simulink model "gm_Model"  (R2025a)
settings: Solver=FixedStepDiscrete  StartTime=0.0  StopTime=80000/fs_in  RelTol=1e-3
undefined symbols (not defined in the file or in its folder): a, b, b_fixp, beta_retanh, c, cos_omega, cos_omega_fixp, diag_count, exp_omega, exp_omega_fixp, fixp_chebacc_frac, fixp_chebacc_ws, fixp_dsp_ws, fixp_eig_frac, fixp_eig_ws, fs_in, group_size, hann_table_fixp, image_seed, image_seed_fixp, J_ROM, k, K_ROM, lap_diags, lap_main, lap_main_fi, lap_offsets, lap_offsets_fi, lap_rest, lap_rest_fi, laplacian_diags_main, laplacian_diags_offsets, laplacian_diags_rest, lut_norm_x, lut_norm_y, magnitude, n_ch, n_layer, n_px, n_px_fi, nf, norm_gain_floor, power_iters, power_norm_scaling_factor_fixp, tau, tau_fixp, theta, theta_fixp
libraries: simulink x59, hdlsllib x36, hdlstreaminglib x4, hdlmdlgenlib x1, matrix_library x1, dspvision x1
(part 6 of 8)

== system gm_Model/DUT_Test/Goertzel/EnabledGoertzel/streaming_partition_streamed1 ==
  in0 : Inport  OutDataTypeStr=fixdt(1, 18, 13)  PortDimensions=[1 48]  SampleTime=3.125e-07
      settings: SignalType=complex
  in1 : Inport  Port=2  OutDataTypeStr=boolean  SampleTime=3.125e-07
  in2 : Inport  Port=3  OutDataTypeStr=fixdt(1, 18, 13)  PortDimensions=[1 48]  SampleTime=3.125e-07
      settings: SignalType=complex
  enb_counter : Inport  Port=4  OutDataTypeStr=uint8  SampleTime=3.125e-07
  Delay3_enbsw : Switch  Criteria=u2 ~= 0  Threshold=double(0)  OutDataTypeStr=fixdt(1, 18, 13)  SampleTime=3.125e-07  SaturateOnIntegerOverflow=off  InputSameDT=off
  Serializer_Subnetwork : Subsystem
  Serializer_Subnetwork1 : Subsystem
  Sum of Elements_out1_bypass : Subsystem
  counter : Subsystem
  enb_counter_eq_97 : simulink/Logic and Bit Operations/Compare To Constant  relop===  const=double(97)  OutDataTypeStr=boolean
  enb_counter_ge_50 : simulink/Logic and Bit Operations/Compare To Constant  relop=>=  const=double(50)  OutDataTypeStr=boolean
  enb_counter_ge_50_and_enb_counter_le_96 : Logic  AllPortsSameDT=off  OutDataTypeStr=boolean  SampleTime=3.125e-07
  enb_counter_le_47 : simulink/Logic and Bit Operations/Compare To Constant  relop=<=  const=double(47)  OutDataTypeStr=boolean
  enb_counter_le_96 : simulink/Logic and Bit Operations/Compare To Constant  relop=<=  const=double(96)  OutDataTypeStr=boolean
  rd_{0..1,3..4,7..8,10..11} (8 alike) : Delay  DelayLength=double(1)  InitialCondition=0  SampleTime=3.125e-07
  rd_12 : Delay  DelayLength=double(6)  InitialCondition=0  SampleTime=3.125e-07
  rd_2 : Delay  DelayLength=double(53)  InitialCondition=0  SampleTime=3.125e-07
  rd_5 : Delay  DelayLength=double(55)  InitialCondition=0  SampleTime=3.125e-07
  rd_6 : Delay  DelayLength=double(54)  InitialCondition=0  SampleTime=3.125e-07
  rd_9 : Delay  DelayLength=double(4)  InitialCondition=0  SampleTime=3.125e-07
  t : Mux  Inputs=2
  tappedDelay : Subsystem
  out0 : Outport  OutDataTypeStr=fixdt(1, 18, 13)  PortDimensions=[1 48]  SampleTime=3.125e-07
      settings: SignalType=complex
  wires:
  rd_3/1 -> Delay3_enbsw/1
  enb_counter/1 -> enb_counter_eq_97/1, enb_counter_le_96/1, enb_counter_ge_50/1, enb_counter_le_47/1
  rd_8/1 -> enb_counter_ge_50_and_enb_counter_le_96/2
  enb_counter_ge_50/1 -> rd_7/1
  enb_counter_le_96/1 -> rd_8/1
  enb_counter_le_47/1 -> rd_1/1
  in0/1 -> rd_0/1
  rd_7/1 -> enb_counter_ge_50_and_enb_counter_le_96/1
  in2/1 -> rd_4/1
  tappedDelay/1(out0) -> rd_10/1
  rd_1/1 -> counter/Enable
  t/1 -> out0/1
  enb_counter_ge_50_and_enb_counter_le_96/1 -> rd_9/1
  rd_5/1 -> Delay3_enbsw/2
  rd_4/1 -> Serializer_Subnetwork1/1(in0)
  counter/1(out0) -> rd_2/1, Serializer_Subnetwork1/2(in1)
  rd_0/1 -> Serializer_Subnetwork/1(in0)
  rd_6/1 -> Delay3_enbsw/3
  rd_2/1 -> Serializer_Subnetwork/2(in1)
  Serializer_Subnetwork/1(out0) -> rd_3/1
  Serializer_Subnetwork1/1(out0) -> rd_6/1
  Delay3_enbsw/1 -> rd_11/1, tappedDelay/1(in0)
  enb_counter_eq_97/1 -> rd_12/1
  rd_12/1 -> Sum of Elements_out1_bypass/2(in1)
  in1/1 -> rd_5/1
  rd_9/1 -> tappedDelay/Enable
  rd_11/1 -> Sum of Elements_out1_bypass/1(in0)
  rd_10/1 -> t/1
  Sum of Elements_out1_bypass/1(out0) -> t/2

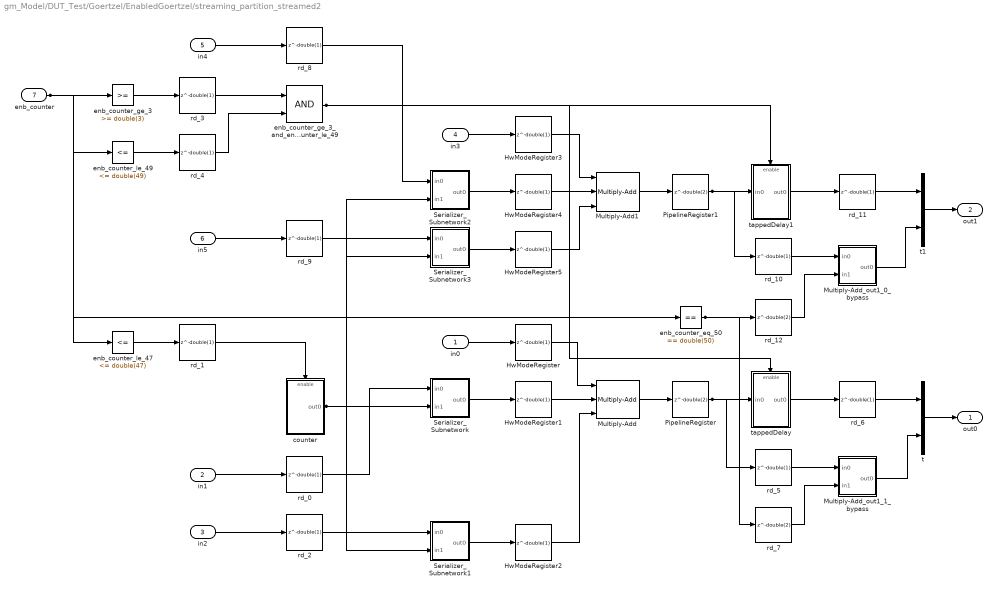
== system gm_Model/DUT_Test/Goertzel/EnabledGoertzel/streaming_partition_streamed2 ==
  in0 : Inport  OutDataTypeStr=fixdt(1, 18, 13)  SampleTime=3.125e-07
      settings: SignalType=complex
  in1 : Inport  Port=2  OutDataTypeStr=fixdt(1, 18, 13)  PortDimensions=[1 48]  SampleTime=3.125e-07
  in2 : Inport  Port=3  OutDataTypeStr=fixdt(1, 18, 13)  PortDimensions=[1 48]  SampleTime=3.125e-07
  in3 : Inport  Port=4  OutDataTypeStr=fixdt(1, 18, 13)  SampleTime=3.125e-07
      settings: SignalType=complex
  in4 : Inport  Port=5  OutDataTypeStr=fixdt(1, 18, 13)  PortDimensions=[1 48]  SampleTime=3.125e-07
  in5 : Inport  Port=6  OutDataTypeStr=fixdt(1, 18, 13)  PortDimensions=[1 48]  SampleTime=3.125e-07
  enb_counter : Inport  Port=7  OutDataTypeStr=uint8  SampleTime=3.125e-07
  HwModeRegister{,1..5} (6 alike) : Delay  DelayLength=double(1)  InitialCondition=0  SampleTime=3.125e-07
  Multiply-Add : hdlsllib/HDL Operations/Multiply-Add  Function=c-(a.*b)  datatype=fixdt(1, 18, 13)  DoSatur=off  FMA=off
  Multiply-Add1 : hdlsllib/HDL Operations/Multiply-Add  Function=c-(a.*b)  datatype=fixdt(1, 18, 13)  DoSatur=off  FMA=off
  Multiply-Add_out1_0_bypass : Subsystem
  Multiply-Add_out1_1_bypass : Subsystem
  PipelineRegister : Delay  DelayLength=double(2)  InitialCondition=0  SampleTime=3.125e-07
  PipelineRegister1 : Delay  DelayLength=double(2)  InitialCondition=0  SampleTime=3.125e-07
  Serializer_Subnetwork : Subsystem
  Serializer_Subnetwork1 : Subsystem
  Serializer_Subnetwork2 : Subsystem
  Serializer_Subnetwork3 : Subsystem
  counter : Subsystem
  enb_counter_eq_50 : simulink/Logic and Bit Operations/Compare To Constant  relop===  const=double(50)  OutDataTypeStr=boolean
  enb_counter_ge_3 : simulink/Logic and Bit Operations/Compare To Constant  relop=>=  const=double(3)  OutDataTypeStr=boolean
  enb_counter_ge_3_and_enb_counter_le_49 : Logic  AllPortsSameDT=off  OutDataTypeStr=boolean  SampleTime=3.125e-07
  enb_counter_le_47 : simulink/Logic and Bit Operations/Compare To Constant  relop=<=  const=double(47)  OutDataTypeStr=boolean
  enb_counter_le_49 : simulink/Logic and Bit Operations/Compare To Constant  relop=<=  const=double(49)  OutDataTypeStr=boolean
  rd_{0..6,8..11} (11 alike) : Delay  DelayLength=double(1)  InitialCondition=0  SampleTime=3.125e-07
  rd_12 : Delay  DelayLength=double(2)  InitialCondition=0  SampleTime=3.125e-07
  rd_7 : Delay  DelayLength=double(2)  InitialCondition=0  SampleTime=3.125e-07
  t : Mux  Inputs=2
  t1 : Mux  Inputs=2
  tappedDelay : Subsystem
  tappedDelay1 : Subsystem
  out0 : Outport  OutDataTypeStr=fixdt(1, 18, 13)  PortDimensions=[1 48]  SampleTime=3.125e-07
      settings: SignalType=complex
  out1 : Outport  Port=2  OutDataTypeStr=fixdt(1, 18, 13)  PortDimensions=[1 48]  SampleTime=3.125e-07
      settings: SignalType=complex
  wires:
  tappedDelay/1(out0) -> rd_6/1
  enb_counter_le_49/1 -> rd_4/1
  HwModeRegister/1 -> Multiply-Add/1
  enb_counter/1 -> enb_counter_le_49/1, enb_counter_ge_3/1, enb_counter_le_47/1, enb_counter_eq_50/1
  rd_4/1 -> enb_counter_ge_3_and_enb_counter_le_49/2
  rd_5/1 -> Multiply-Add_out1_1_bypass/1(in0)
  Serializer_Subnetwork3/1(out0) -> HwModeRegister5/1
  in1/1 -> rd_0/1
  rd_3/1 -> enb_counter_ge_3_and_enb_counter_le_49/1
  enb_counter_ge_3/1 -> rd_3/1
  enb_counter_le_47/1 -> rd_1/1
  rd_12/1 -> Multiply-Add_out1_0_bypass/2(in1)
  in5/1 -> rd_9/1
  in4/1 -> rd_8/1
  rd_1/1 -> counter/Enable
  in2/1 -> rd_2/1
  rd_8/1 -> Serializer_Subnetwork2/1(in0)
  enb_counter_ge_3_and_enb_counter_le_49/1 -> tappedDelay1/Enable, tappedDelay/Enable
  rd_2/1 -> Serializer_Subnetwork1/1(in0)
  rd_9/1 -> Serializer_Subnetwork3/1(in0)
  counter/1(out0) -> Serializer_Subnetwork3/2(in1), Serializer_Subnetwork2/2(in1), Serializer_Subnetwork1/2(in1), Serializer_Subnetwork/2(in1)
  in0/1 -> HwModeRegister/1
  rd_0/1 -> Serializer_Subnetwork/1(in0)
  in3/1 -> HwModeRegister3/1
  Serializer_Subnetwork2/1(out0) -> HwModeRegister4/1
  Serializer_Subnetwork/1(out0) -> HwModeRegister1/1
  HwModeRegister5/1 -> Multiply-Add1/3
  HwModeRegister3/1 -> Multiply-Add1/1
  Serializer_Subnetwork1/1(out0) -> HwModeRegister2/1
  HwModeRegister4/1 -> Multiply-Add1/2
  PipelineRegister1/1 -> rd_10/1, tappedDelay1/1(in0)
  Multiply-Add/1 -> PipelineRegister/1
  HwModeRegister1/1 -> Multiply-Add/2
  HwModeRegister2/1 -> Multiply-Add/3
  Multiply-Add1/1 -> PipelineRegister1/1
  Multiply-Add_out1_1_bypass/1(out0) -> t/2
  enb_counter_eq_50/1 -> rd_7/1, rd_12/1
  PipelineRegister/1 -> rd_5/1, tappedDelay/1(in0)
  tappedDelay1/1(out0) -> rd_11/1
  rd_10/1 -> Multiply-Add_out1_0_bypass/1(in0)
  rd_7/1 -> Multiply-Add_out1_1_bypass/2(in1)
  rd_6/1 -> t/1
  rd_11/1 -> t1/1
  Multiply-Add_out1_0_bypass/1(out0) -> t1/2
  t1/1 -> out1/1
  t/1 -> out0/1

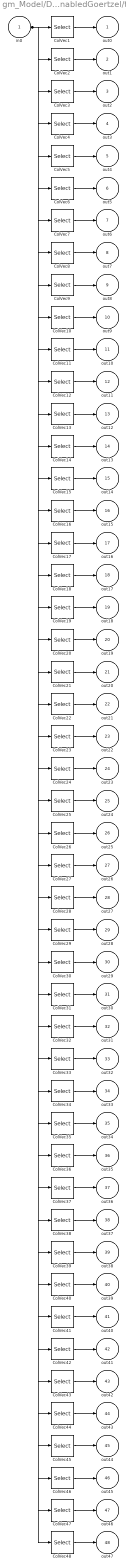
== system gm_Model/DUT_Test/Goertzel/EnabledGoertzel/t2 ==
  in0 : Inport
  ColVec1 : Selector  NumberOfDimensions=2  IndexOptions=Select all,Index vector (dialog)  Indices=1,1  OutputSizes=1,1
  ColVec10 : Selector  NumberOfDimensions=2  IndexOptions=Select all,Index vector (dialog)  Indices=1,10  OutputSizes=1,1
  ColVec11 : Selector  NumberOfDimensions=2  IndexOptions=Select all,Index vector (dialog)  Indices=1,11  OutputSizes=1,1
  ColVec12 : Selector  NumberOfDimensions=2  IndexOptions=Select all,Index vector (dialog)  Indices=1,12  OutputSizes=1,1
  ColVec13 : Selector  NumberOfDimensions=2  IndexOptions=Select all,Index vector (dialog)  Indices=1,13  OutputSizes=1,1
  ColVec14 : Selector  NumberOfDimensions=2  IndexOptions=Select all,Index vector (dialog)  Indices=1,14  OutputSizes=1,1
  ColVec15 : Selector  NumberOfDimensions=2  IndexOptions=Select all,Index vector (dialog)  Indices=1,15  OutputSizes=1,1
  ColVec16 : Selector  NumberOfDimensions=2  IndexOptions=Select all,Index vector (dialog)  Indices=1,16  OutputSizes=1,1
  ColVec17 : Selector  NumberOfDimensions=2  IndexOptions=Select all,Index vector (dialog)  Indices=1,17  OutputSizes=1,1
  ColVec18 : Selector  NumberOfDimensions=2  IndexOptions=Select all,Index vector (dialog)  Indices=1,18  OutputSizes=1,1
  ColVec19 : Selector  NumberOfDimensions=2  IndexOptions=Select all,Index vector (dialog)  Indices=1,19  OutputSizes=1,1
  ColVec2 : Selector  NumberOfDimensions=2  IndexOptions=Select all,Index vector (dialog)  Indices=1,2  OutputSizes=1,1
  ColVec20 : Selector  NumberOfDimensions=2  IndexOptions=Select all,Index vector (dialog)  Indices=1,20  OutputSizes=1,1
  ColVec21 : Selector  NumberOfDimensions=2  IndexOptions=Select all,Index vector (dialog)  Indices=1,21  OutputSizes=1,1
  ColVec22 : Selector  NumberOfDimensions=2  IndexOptions=Select all,Index vector (dialog)  Indices=1,22  OutputSizes=1,1
  ColVec23 : Selector  NumberOfDimensions=2  IndexOptions=Select all,Index vector (dialog)  Indices=1,23  OutputSizes=1,1
  ColVec24 : Selector  NumberOfDimensions=2  IndexOptions=Select all,Index vector (dialog)  Indices=1,24  OutputSizes=1,1
  ColVec25 : Selector  NumberOfDimensions=2  IndexOptions=Select all,Index vector (dialog)  Indices=1,25  OutputSizes=1,1
  ColVec26 : Selector  NumberOfDimensions=2  IndexOptions=Select all,Index vector (dialog)  Indices=1,26  OutputSizes=1,1
  ColVec27 : Selector  NumberOfDimensions=2  IndexOptions=Select all,Index vector (dialog)  Indices=1,27  OutputSizes=1,1
  ColVec28 : Selector  NumberOfDimensions=2  IndexOptions=Select all,Index vector (dialog)  Indices=1,28  OutputSizes=1,1
  ColVec29 : Selector  NumberOfDimensions=2  IndexOptions=Select all,Index vector (dialog)  Indices=1,29  OutputSizes=1,1
  ColVec3 : Selector  NumberOfDimensions=2  IndexOptions=Select all,Index vector (dialog)  Indices=1,3  OutputSizes=1,1
  ColVec30 : Selector  NumberOfDimensions=2  IndexOptions=Select all,Index vector (dialog)  Indices=1,30  OutputSizes=1,1
  ColVec31 : Selector  NumberOfDimensions=2  IndexOptions=Select all,Index vector (dialog)  Indices=1,31  OutputSizes=1,1
  ColVec32 : Selector  NumberOfDimensions=2  IndexOptions=Select all,Index vector (dialog)  Indices=1,32  OutputSizes=1,1
  ColVec33 : Selector  NumberOfDimensions=2  IndexOptions=Select all,Index vector (dialog)  Indices=1,33  OutputSizes=1,1
  ColVec34 : Selector  NumberOfDimensions=2  IndexOptions=Select all,Index vector (dialog)  Indices=1,34  OutputSizes=1,1
  ColVec35 : Selector  NumberOfDimensions=2  IndexOptions=Select all,Index vector (dialog)  Indices=1,35  OutputSizes=1,1
  ColVec36 : Selector  NumberOfDimensions=2  IndexOptions=Select all,Index vector (dialog)  Indices=1,36  OutputSizes=1,1
  ColVec37 : Selector  NumberOfDimensions=2  IndexOptions=Select all,Index vector (dialog)  Indices=1,37  OutputSizes=1,1
  ColVec38 : Selector  NumberOfDimensions=2  IndexOptions=Select all,Index vector (dialog)  Indices=1,38  OutputSizes=1,1
  ColVec39 : Selector  NumberOfDimensions=2  IndexOptions=Select all,Index vector (dialog)  Indices=1,39  OutputSizes=1,1
  ColVec4 : Selector  NumberOfDimensions=2  IndexOptions=Select all,Index vector (dialog)  Indices=1,4  OutputSizes=1,1
  ColVec40 : Selector  NumberOfDimensions=2  IndexOptions=Select all,Index vector (dialog)  Indices=1,40  OutputSizes=1,1
  ColVec41 : Selector  NumberOfDimensions=2  IndexOptions=Select all,Index vector (dialog)  Indices=1,41  OutputSizes=1,1
  ColVec42 : Selector  NumberOfDimensions=2  IndexOptions=Select all,Index vector (dialog)  Indices=1,42  OutputSizes=1,1
  ColVec43 : Selector  NumberOfDimensions=2  IndexOptions=Select all,Index vector (dialog)  Indices=1,43  OutputSizes=1,1
  ColVec44 : Selector  NumberOfDimensions=2  IndexOptions=Select all,Index vector (dialog)  Indices=1,44  OutputSizes=1,1
  ColVec45 : Selector  NumberOfDimensions=2  IndexOptions=Select all,Index vector (dialog)  Indices=1,45  OutputSizes=1,1
  ColVec46 : Selector  NumberOfDimensions=2  IndexOptions=Select all,Index vector (dialog)  Indices=1,46  OutputSizes=1,1
  ColVec47 : Selector  NumberOfDimensions=2  IndexOptions=Select all,Index vector (dialog)  Indices=1,47  OutputSizes=1,1
  ColVec48 : Selector  NumberOfDimensions=2  IndexOptions=Select all,Index vector (dialog)  Indices=1,48  OutputSizes=1,1
  ColVec5 : Selector  NumberOfDimensions=2  IndexOptions=Select all,Index vector (dialog)  Indices=1,5  OutputSizes=1,1
  ColVec6 : Selector  NumberOfDimensions=2  IndexOptions=Select all,Index vector (dialog)  Indices=1,6  OutputSizes=1,1
  ColVec7 : Selector  NumberOfDimensions=2  IndexOptions=Select all,Index vector (dialog)  Indices=1,7  OutputSizes=1,1
  ColVec8 : Selector  NumberOfDimensions=2  IndexOptions=Select all,Index vector (dialog)  Indices=1,8  OutputSizes=1,1
  ColVec9 : Selector  NumberOfDimensions=2  IndexOptions=Select all,Index vector (dialog)  Indices=1,9  OutputSizes=1,1
  out0 : Outport
  out1 : Outport  Port=2
  out2 : Outport  Port=3
  out3 : Outport  Port=4
  out4 : Outport  Port=5
  out5 : Outport  Port=6
  out6 : Outport  Port=7
  out7 : Outport  Port=8
  out8 : Outport  Port=9
  out9 : Outport  Port=10
  out10 : Outport  Port=11
  out11 : Outport  Port=12
  out12 : Outport  Port=13
  out13 : Outport  Port=14
  out14 : Outport  Port=15
  out15 : Outport  Port=16
  out16 : Outport  Port=17
  out17 : Outport  Port=18
  out18 : Outport  Port=19
  out19 : Outport  Port=20
  out20 : Outport  Port=21
  out21 : Outport  Port=22
  out22 : Outport  Port=23
  out23 : Outport  Port=24
  out24 : Outport  Port=25
  out25 : Outport  Port=26
  out26 : Outport  Port=27
  out27 : Outport  Port=28
  out28 : Outport  Port=29
  out29 : Outport  Port=30
  out30 : Outport  Port=31
  out31 : Outport  Port=32
  out32 : Outport  Port=33
  out33 : Outport  Port=34
  out34 : Outport  Port=35
  out35 : Outport  Port=36
  out36 : Outport  Port=37
  out37 : Outport  Port=38
  out38 : Outport  Port=39
  out39 : Outport  Port=40
  out40 : Outport  Port=41
  out41 : Outport  Port=42
  out42 : Outport  Port=43
  out43 : Outport  Port=44
  out44 : Outport  Port=45
  out45 : Outport  Port=46
  out46 : Outport  Port=47
  out47 : Outport  Port=48
  wires:
  in0/1 -> ColVec1/1, ColVec2/1, ColVec3/1, ColVec4/1, ColVec5/1, ColVec6/1, ColVec7/1, ColVec8/1, ColVec9/1, ColVec10/1, ColVec11/1, ColVec12/1, ColVec13/1, ColVec14/1, ColVec15/1, ColVec16/1, ColVec17/1, ColVec18/1, ColVec19/1, ColVec20/1, ColVec21/1, ColVec22/1, ColVec23/1, ColVec24/1, ColVec25/1, ColVec26/1, ColVec27/1, ColVec28/1, ColVec29/1, ColVec30/1, ColVec31/1, ColVec32/1, ColVec33/1, ColVec34/1, ColVec35/1, ColVec36/1, ColVec37/1, ColVec38/1, ColVec39/1, ColVec40/1, ColVec41/1, ColVec42/1, ColVec43/1, ColVec44/1, ColVec45/1, ColVec46/1, ColVec47/1, ColVec48/1
  ColVec1/1 -> out0/1
  ColVec2/1 -> out1/1
  ColVec3/1 -> out2/1
  ColVec4/1 -> out3/1
  ColVec5/1 -> out4/1
  ColVec6/1 -> out5/1
  ColVec7/1 -> out6/1
  ColVec8/1 -> out7/1
  ColVec9/1 -> out8/1
  ColVec10/1 -> out9/1
  ColVec11/1 -> out10/1
  ColVec12/1 -> out11/1
  ColVec13/1 -> out12/1
  ColVec14/1 -> out13/1
  ColVec15/1 -> out14/1
  ColVec16/1 -> out15/1
  ColVec17/1 -> out16/1
  ColVec18/1 -> out17/1
  ColVec19/1 -> out18/1
  ColVec20/1 -> out19/1
  ColVec21/1 -> out20/1
  ColVec22/1 -> out21/1
  ColVec23/1 -> out22/1
  ColVec24/1 -> out23/1
  ColVec25/1 -> out24/1
  ColVec26/1 -> out25/1
  ColVec27/1 -> out26/1
  ColVec28/1 -> out27/1
  ColVec29/1 -> out28/1
  ColVec30/1 -> out29/1
  ColVec31/1 -> out30/1
  ColVec32/1 -> out31/1
  ColVec33/1 -> out32/1
  ColVec34/1 -> out33/1
  ColVec35/1 -> out34/1
  ColVec36/1 -> out35/1
  ColVec37/1 -> out36/1
  ColVec38/1 -> out37/1
  ColVec39/1 -> out38/1
  ColVec40/1 -> out39/1
  ColVec41/1 -> out40/1
  ColVec42/1 -> out41/1
  ColVec43/1 -> out42/1
  ColVec44/1 -> out43/1
  ColVec45/1 -> out44/1
  ColVec46/1 -> out45/1
  ColVec47/1 -> out46/1
  ColVec48/1 -> out47/1

== system gm_Model/DUT_ref/CrossCor/Grouping/DataValidDownsampler ==
  ValidFast : Inport
  DataFast : Inport  Port=2
  DataInSW : Switch  Criteria=u2 ~= 0  SaturateOnIntegerOverflow=off  InputSameDT=off
  DataMem : Delay  DelayLength=1
  DataRT : RateTransition  Deterministic=off  OutPortSampleTimeOpt=Multiple of input port sample time  OutPortSampleTimeMultiple=rate_factor
  RisingEdgeDetector : Subsystem
  Terminator : Terminator
  ValidMem : Delay  DelayLength=1  ShowEnablePort=on
      settings: InputPortMap=u0,e6
  ValidRT : RateTransition  Deterministic=off  OutPortSampleTimeOpt=Multiple of input port sample time  OutPortSampleTimeMultiple=rate_factor
  ValidResetCounter : hdlsllib/Sources/HDL Counter  CountType=Count limited  CountInit=0  CountStep=1  CountMax=rate_factor-1  CountFromType=Initial value  CountFrom=0  CountResetPort=off  CountLoadPort=off  CountEnbPort=off  CountDirPort=off  CountHitOutputPort=on  CountDataType=Unsigned  CountWordLen=ceil(log2(rate_factor))  CountFracLen=0  CountSampTime=-1
  ValidResetDelay : Delay  DelayLength=1
  ValidSampleOR : Logic  Operator=OR  IconShape=distinctive  AllPortsSameDT=off  OutDataTypeStr=boolean
  ValidSlow : Outport
  DataSlow : Outport  Port=2
  wires:
  ValidResetCounter/1 -> Terminator/1
  DataFast/1 -> DataInSW/1
  DataRT/1 -> DataSlow/1
  ValidRT/1 -> ValidSlow/1
  ValidMem/1 -> ValidRT/1
  ValidResetDelay/1 -> ValidSampleOR/2
  ValidResetCounter/2 -> ValidResetDelay/1
  ValidFast/1 -> RisingEdgeDetector/1(In1)
  RisingEdgeDetector/1(Out1) -> ValidMem/1, ValidSampleOR/1, DataInSW/2
  DataInSW/1 -> DataMem/1
  DataMem/1 -> DataInSW/3, DataRT/1
  ValidSampleOR/1 -> ValidMem/2

== system gm_Model/DUT_ref/CrossCor/NormalizationEigen/PowerIteration ==
  note: Norm of vector: sum(sq(abs(v)))
  MatIn : Inport
  Compare To Constant : simulink/Logic and Bit Operations/Compare To Constant  relop=<=  const=1e-8  OutDataTypeStr=boolean
  Complex to Real-Imag : ComplexToRealImag  Output=Real
  Delay : Delay  DelayLength=1  InitialCondition=0
  Delay1 : Delay  DelayLength=1
  Delay2 : Delay  DelayLength=1  InitialCondition=0
  Divide : Product  Inputs=**
  HDL Counter : hdlsllib/Sources/HDL Counter  CountType=Count limited  CountInit=0  CountStep=1  CountMax=power_iters-1  CountFromType=Initial value  CountFrom=0  CountResetPort=off  CountLoadPort=off  CountEnbPort=off  CountDirPort=off  CountHitOutputPort=off  CountDataType=Unsigned  CountWordLen=6  CountFracLen=0  CountSampTime=group_size*nf/(fs_in*power_iters)
  Hermitian : Math  Operator=hermitian
  Matrix Multiply : Product  Multiplication=Matrix(*)
  Matrix Multiply1 : Product  Multiplication=Matrix(*)
  Matrix Multiply2 : Product  Multiplication=Matrix(*)
  One : Constant  OutDataTypeStr=Inherit: Inherit via back propagation  SampleTime=-1
  Product : Product
  Rate Transition : RateTransition  InitialCondition=1
  Rate Transition1 : RateTransition  Integrity=off  OutPortSampleTimeOpt=Multiple of input port sample time  OutPortSampleTimeMultiple=1/power_iters
  Rate Transition2 : RateTransition  InitialCondition=1
  Real-Imag to Complex : RealImagToComplex  Input=Real
  Reciprocal : Product  Inputs=/
  SeedEigenVec : Constant  Value=ones(1,n_ch)'./sqrt(n_ch)  VectorParams1D=off  OutDataTypeStr=Inherit: Inherit via back propagation  SampleTime=-1
  Square : Math  Operator=magnitude^2
  Sum of Elements : Sum  Inputs=+
  Switch : Switch  Criteria=u2 > Threshold  SaturateOnIntegerOverflow=off  InputSameDT=off
  Switch1 : Switch  Criteria=u2 ~= 0  SaturateOnIntegerOverflow=off  InputSameDT=off
  MatOut : Outport
  MaxEigenvalue : Outport  Port=2
  wires:
  Reciprocal/1 -> Divide/2
  Switch1/1 -> Reciprocal/1, Delay2/1
  Rate Transition2/1 -> Product/2  "Norm"
  Delay2/1 -> Rate Transition2/1
  Product/1 -> MaxEigenvalue/1
  Complex to Real-Imag/1 -> Product/1
  Compare To Constant/1 -> Switch1/2
  One/1 -> Switch1/1
  Sum of Elements/1 -> Compare To Constant/1, Switch1/3
  Matrix Multiply1/1 -> Matrix Multiply2/1
  Hermitian/1 -> Matrix Multiply1/1
  Real-Imag to Complex/1 -> Switch/3
  SeedEigenVec/1 -> Real-Imag to Complex/1
  Delay1/1 -> MatOut/1, Matrix Multiply1/2
  Matrix Multiply2/1 -> Complex to Real-Imag/1
  Square/1 -> Sum of Elements/1
  Divide/1 -> Delay/1
  MatIn/1 -> Rate Transition1/1, Delay1/1
  Rate Transition1/1 -> Matrix Multiply/1
  Matrix Multiply/1 -> Divide/1, Square/1
  HDL Counter/1 -> Switch/2
  Switch/1 -> Matrix Multiply/2
  Rate Transition/1 -> Hermitian/1, Matrix Multiply2/2
  Delay/1 -> Rate Transition/1, Switch/1

== system gm_Model/DUT_ref/Deblurring/Chebyshev/AccumulatorCounter ==
  a : Inport
  b : Inport  Port=2
  Delay : Delay  DelayLength=1
  Delay1 : Delay  DelayLength=1
  HDL Counter : hdlsllib/Sources/HDL Counter  CountType=Count limited  CountInit=0  CountStep=1  CountMax=k  CountFromType=Initial value  CountFrom=0  CountResetPort=off  CountLoadPort=off  CountEnbPort=off  CountDirPort=off  CountHitOutputPort=on  CountDataType=Unsigned  CountWordLen=8  CountFracLen=0  CountSampTime=-1
  Multiply-Add : hdlsllib/HDL Operations/Multiply-Add  Function=c+(a.*b)  datatype=Inherit: Inherit via internal rule  DoSatur=off  FMA=off
  Switch : Switch  Criteria=u2 ~= 0  SaturateOnIntegerOverflow=off  InputSameDT=off
  Zero : Constant  Value=0  OutDataTypeStr=Inherit: Inherit via back propagation  SampleTime=-1
  counter : Outport
  accum : Outport  Port=2
  wires:
  Switch/1 -> Multiply-Add/3
  Delay/1 -> accum/1, Switch/3
  Multiply-Add/1 -> Delay/1
  Delay1/1 -> Switch/2
  Zero/1 -> Switch/1
  HDL Counter/1 -> counter/1
  b/1 -> Multiply-Add/2
  a/1 -> Multiply-Add/1
  HDL Counter/2 -> Delay1/1

== system gm_Model/DUT_ref/Deblurring/Chebyshev/LaplacianMultiply ==
  Image_in : Inport
  Constant : Constant  Value=lap_diags
  Constant1 : Constant  Value=lap_offsets
  Delay : Delay  DelayLength=1
  For Each Subsystem : Subsystem  TreatAsAtomicUnit=on
  Image_out : Outport
  wires:
  Delay/1 -> For Each Subsystem/1(ToIterate), For Each Subsystem/2(Image)
  Image_in/1 -> Delay/1
  Constant1/1 -> For Each Subsystem/4(Offset)
  For Each Subsystem/1(Image_out) -> Image_out/1
  Constant/1 -> For Each Subsystem/3(Diag)

== system gm_Model/DUT_ref/Goertzel/DataValidDownsampler/RisingEdgeDetector ==
  In1 : Inport
  AND : Logic  IconShape=distinctive  AllPortsSameDT=off  OutDataTypeStr=boolean
  Delay1 : Delay  DelayLength=1
  NOT : Logic  Operator=NOT  IconShape=distinctive  AllPortsSameDT=off  OutDataTypeStr=boolean
  Out1 : Outport
  wires:
  Delay1/1 -> NOT/1
  AND/1 -> Out1/1
  NOT/1 -> AND/1
  In1/1 -> AND/2, Delay1/1

== system gm_Model/DUT_ref/Goertzel/EnabledGoertzel/Goertzel filter ==
  u : Inport
  Reset : ResetPort  DisableCoverage=on  ResetTriggerType=level hold
  Complex to Real-Imag : ComplexToRealImag  Commented=on
  For All Bins Filter : Subsystem  TreatAsAtomicUnit=on  mask{cos_omega=cos_omega, exp_omega=exp_omega}
  GoertzelImMax : MinMax  Commented=on  Function=max
  GoertzelImMin : MinMax  Commented=on
  GoertzelReMax : MinMax  Commented=on  Function=max
  GoertzelReMin : MinMax  Commented=on
  State Control : StateControl  StateControl=Synchronous
  Sum of Elements : Sum  Inputs=+  CollapseMode=Specified dimension
  Out1 : Outport  VectorParamsAs1DForOutWhenUnconnected=off
  wires:
  For All Bins Filter/1(Out1) -> Sum of Elements/1, Complex to Real-Imag/1
  Complex to Real-Imag/2 -> GoertzelImMin/1, GoertzelImMax/1
  Complex to Real-Imag/1 -> GoertzelReMax/1, GoertzelReMin/1
  Sum of Elements/1 -> Out1/1
  u/1 -> For All Bins Filter/1(In1)

== system gm_Model/DUT_ref/Goertzel/EnabledGoertzel/Symmetric Hann ==
  u : Inport
  Compare To Constant : simulink/Logic and Bit Operations/Compare To Constant  relop=<  const=nf/2  OutDataTypeStr=boolean
  Constant : Constant  Value=nf-1
  Hann : Lookup_n-D  NumberOfTableDimensions=1  LookupTableObject=''  BreakpointsSpecification=Even spacing  BreakpointsForDimension1=[1:200]  BreakpointsForDimension1FirstPoint=0  BreakpointsForDimension2FirstPoint=10  BreakpointsForDimension2Spacing=12  IndexSearchMethod=Evenly spaced points  Table=0.5*(1-cos(2*pi*[0:(nf/2-1)]/(nf-1)))  InterpMethod=Flat  DiagnosticForOutOfRangeInput=Error  InternalRulePriority=Speed  RndMeth=Simplest
  Sum : Sum  Inputs=|-+
  Switch : Switch  Criteria=u2 ~= 0  SaturateOnIntegerOverflow=off  InputSameDT=off
  Out1 : Outport
  wires:
  Hann/1 -> Out1/1
  Compare To Constant/1 -> Switch/2
  Switch/1 -> Hann/1
  Constant/1 -> Sum/2
  Sum/1 -> Switch/3
  u/1 -> Sum/1, Compare To Constant/1, Switch/1

== system gm_Model/DUT_FixP/CrossCor/Grouping/DataValidDownsampler/RisingEdgeDetector ==
  In1 : Inport
  AND : Logic  IconShape=distinctive  AllPortsSameDT=off  OutDataTypeStr=boolean
  Delay1 : Delay  DelayLength=1
  NOT : Logic  Operator=NOT  IconShape=distinctive  AllPortsSameDT=off  OutDataTypeStr=boolean
  Out1 : Outport
  wires:
  Delay1/1 -> NOT/1
  AND/1 -> Out1/1
  NOT/1 -> AND/1
  In1/1 -> AND/2, Delay1/1

== system gm_Model/DUT_FixP/Goertzel/EnabledGoertzel/Goertzel filter/For All Bins Filter ==
  In : Inport
  Reset : Inport  Port=2
  Constant : Constant  Value=0  OutDataTypeStr=Inherit: Inherit via back propagation  SampleTime=-1
  Constant1 : Constant  Value=0  OutDataTypeStr=Inherit: Inherit via back propagation  SampleTime=-1
  Cos_omega_mult : Gain  Gain=cos_omega  ParamDataTypeStr=Inherit: Inherit from 'Gain'  OutDataTypeStr=Inherit: Same as input
  Delay : Delay  DelayLength=1
  Delay1 : Delay  DelayLength=1
  Exp_omega_mult : Gain  Gain=exp_omega  ParamDataTypeStr=Inherit: Inherit from 'Gain'  OutDataTypeStr=Inherit: Same as input
  For Each : ForEach  DisableCoverage=on  IterateSubsysMaskParameter=on,on  SubsysMaskParameterIterationDimension=2,2
  Sum : Sum  Inputs=++-  OutDataTypeStr=Inherit: Same as accumulator  AccumDataTypeStr=fixdt(1,fixp_input_ws+fixp_goertzel_int_bits+2,fixp_input_ws+2-1)
  Sum1 : Sum  Inputs=|-+  OutDataTypeStr=Inherit: Same as accumulator
  Switch : Switch  Criteria=u2 ~= 0  SaturateOnIntegerOverflow=off  InputSameDT=off
  Switch1 : Switch  Criteria=u2 ~= 0  SaturateOnIntegerOverflow=off  InputSameDT=off
  Out1 : Outport  ConcatenationDimension=1
  wires:
  Switch1/1 -> Delay1/1
  Constant1/1 -> Switch1/1
  Sum/1 -> Switch1/3
  Switch/1 -> Delay/1
  Constant/1 -> Switch/1
  Reset/1 -> Switch/2, Switch1/2
  Delay/1 -> Sum1/2, Sum/3
  Delay1/1 -> Cos_omega_mult/1, Exp_omega_mult/1, Switch/3
  Exp_omega_mult/1 -> Sum1/1
  Cos_omega_mult/1 -> Sum/1
  Sum1/1 -> Out1/1
  In/1 -> Sum/2

== system gm_Model/DUT_Test/Goertzel/EnabledGoertzel/crp_temp_streamed/Serializer_Subnetwork ==
  in0 : Inport  OutDataTypeStr=fixdt(1, 12, 11)  PortDimensions=[1 48]  SampleTime=3.125e-07
  in1 : Inport  Port=2  OutDataTypeStr=fixdt(0, 6, 0)  SampleTime=3.125e-07
  ratechange_splitcomp : Demux  Outputs=48
  splitcomp_multiport : MultiPortSwitch  DataPortOrder=Zero-based contiguous  Inputs=48  DiagnosticForDefault=None  zeroidx=on  OutDataTypeStr=fixdt(1, 12, 11)  SampleTime=3.125e-07  SaturateOnIntegerOverflow=off  InputSameDT=off
  out0 : Outport  OutDataTypeStr=fixdt(1, 12, 11)  SampleTime=3.125e-07
  wires:
  in0/1 -> ratechange_splitcomp/1
  in1/1 -> splitcomp_multiport/1
  ratechange_splitcomp/1 -> splitcomp_multiport/2
  ratechange_splitcomp/2 -> splitcomp_multiport/3
  ratechange_splitcomp/3 -> splitcomp_multiport/4
  ratechange_splitcomp/7 -> splitcomp_multiport/8
  ratechange_splitcomp/4 -> splitcomp_multiport/5
  ratechange_splitcomp/5 -> splitcomp_multiport/6
  ratechange_splitcomp/6 -> splitcomp_multiport/7
  ratechange_splitcomp/11 -> splitcomp_multiport/12
  ratechange_splitcomp/10 -> splitcomp_multiport/11
  ratechange_splitcomp/9 -> splitcomp_multiport/10
  ratechange_splitcomp/8 -> splitcomp_multiport/9
  ratechange_splitcomp/15 -> splitcomp_multiport/16
  ratechange_splitcomp/14 -> splitcomp_multiport/15
  ratechange_splitcomp/13 -> splitcomp_multiport/14
  ratechange_splitcomp/12 -> splitcomp_multiport/13
  ratechange_splitcomp/19 -> splitcomp_multiport/20
  ratechange_splitcomp/18 -> splitcomp_multiport/19
  ratechange_splitcomp/17 -> splitcomp_multiport/18
  ratechange_splitcomp/16 -> splitcomp_multiport/17
  ratechange_splitcomp/23 -> splitcomp_multiport/24
  ratechange_splitcomp/22 -> splitcomp_multiport/23
  ratechange_splitcomp/21 -> splitcomp_multiport/22
  ratechange_splitcomp/20 -> splitcomp_multiport/21
  ratechange_splitcomp/27 -> splitcomp_multiport/28
  ratechange_splitcomp/26 -> splitcomp_multiport/27
  ratechange_splitcomp/25 -> splitcomp_multiport/26
  ratechange_splitcomp/24 -> splitcomp_multiport/25
  ratechange_splitcomp/31 -> splitcomp_multiport/32
  ratechange_splitcomp/30 -> splitcomp_multiport/31
  ratechange_splitcomp/29 -> splitcomp_multiport/30
  ratechange_splitcomp/28 -> splitcomp_multiport/29
  ratechange_splitcomp/35 -> splitcomp_multiport/36
  ratechange_splitcomp/34 -> splitcomp_multiport/35
  ratechange_splitcomp/33 -> splitcomp_multiport/34
  ratechange_splitcomp/32 -> splitcomp_multiport/33
  ratechange_splitcomp/39 -> splitcomp_multiport/40
  ratechange_splitcomp/38 -> splitcomp_multiport/39
  ratechange_splitcomp/37 -> splitcomp_multiport/38
  ratechange_splitcomp/36 -> splitcomp_multiport/37
  ratechange_splitcomp/43 -> splitcomp_multiport/44
  ratechange_splitcomp/42 -> splitcomp_multiport/43
  ratechange_splitcomp/41 -> splitcomp_multiport/42
  ratechange_splitcomp/40 -> splitcomp_multiport/41
  ratechange_splitcomp/47 -> splitcomp_multiport/48
  ratechange_splitcomp/46 -> splitcomp_multiport/47
  ratechange_splitcomp/45 -> splitcomp_multiport/46
  ratechange_splitcomp/44 -> splitcomp_multiport/45
  ratechange_splitcomp/48 -> splitcomp_multiport/49
  splitcomp_multiport/1 -> out0/1

== system gm_Model/DUT_Test/Goertzel/EnabledGoertzel/crp_temp_streamed/Serializer_Subnetwork1 ==
  in0 : Inport  OutDataTypeStr=fixdt(1, 12, 11)  PortDimensions=[1 48]  SampleTime=3.125e-07
  in1 : Inport  Port=2  OutDataTypeStr=fixdt(0, 6, 0)  SampleTime=3.125e-07
  ratechange_splitcomp : Demux  Outputs=48
  splitcomp_multiport : MultiPortSwitch  DataPortOrder=Zero-based contiguous  Inputs=48  DiagnosticForDefault=None  zeroidx=on  OutDataTypeStr=fixdt(1, 12, 11)  SampleTime=3.125e-07  SaturateOnIntegerOverflow=off  InputSameDT=off
  out0 : Outport  OutDataTypeStr=fixdt(1, 12, 11)  SampleTime=3.125e-07
  wires:
  in0/1 -> ratechange_splitcomp/1
  in1/1 -> splitcomp_multiport/1
  ratechange_splitcomp/1 -> splitcomp_multiport/2
  ratechange_splitcomp/2 -> splitcomp_multiport/3
  ratechange_splitcomp/3 -> splitcomp_multiport/4
  ratechange_splitcomp/4 -> splitcomp_multiport/5
  ratechange_splitcomp/8 -> splitcomp_multiport/9
  ratechange_splitcomp/7 -> splitcomp_multiport/8
  ratechange_splitcomp/5 -> splitcomp_multiport/6
  ratechange_splitcomp/6 -> splitcomp_multiport/7
  ratechange_splitcomp/12 -> splitcomp_multiport/13
  ratechange_splitcomp/11 -> splitcomp_multiport/12
  ratechange_splitcomp/10 -> splitcomp_multiport/11
  ratechange_splitcomp/9 -> splitcomp_multiport/10
  ratechange_splitcomp/16 -> splitcomp_multiport/17
  ratechange_splitcomp/15 -> splitcomp_multiport/16
  ratechange_splitcomp/14 -> splitcomp_multiport/15
  ratechange_splitcomp/13 -> splitcomp_multiport/14
  ratechange_splitcomp/40 -> splitcomp_multiport/41
  ratechange_splitcomp/20 -> splitcomp_multiport/21
  ratechange_splitcomp/19 -> splitcomp_multiport/20
  ratechange_splitcomp/18 -> splitcomp_multiport/19
  ratechange_splitcomp/17 -> splitcomp_multiport/18
  ratechange_splitcomp/24 -> splitcomp_multiport/25
  ratechange_splitcomp/23 -> splitcomp_multiport/24
  ratechange_splitcomp/22 -> splitcomp_multiport/23
  ratechange_splitcomp/21 -> splitcomp_multiport/22
  ratechange_splitcomp/28 -> splitcomp_multiport/29
  ratechange_splitcomp/27 -> splitcomp_multiport/28
  ratechange_splitcomp/26 -> splitcomp_multiport/27
  ratechange_splitcomp/25 -> splitcomp_multiport/26
  ratechange_splitcomp/32 -> splitcomp_multiport/33
  ratechange_splitcomp/31 -> splitcomp_multiport/32
  ratechange_splitcomp/30 -> splitcomp_multiport/31
  ratechange_splitcomp/29 -> splitcomp_multiport/30
  ratechange_splitcomp/36 -> splitcomp_multiport/37
  ratechange_splitcomp/35 -> splitcomp_multiport/36
  ratechange_splitcomp/34 -> splitcomp_multiport/35
  ratechange_splitcomp/33 -> splitcomp_multiport/34
  ratechange_splitcomp/39 -> splitcomp_multiport/40
  ratechange_splitcomp/38 -> splitcomp_multiport/39
  ratechange_splitcomp/37 -> splitcomp_multiport/38
  ratechange_splitcomp/41 -> splitcomp_multiport/42
  ratechange_splitcomp/45 -> splitcomp_multiport/46
  ratechange_splitcomp/44 -> splitcomp_multiport/45
  ratechange_splitcomp/43 -> splitcomp_multiport/44
  ratechange_splitcomp/42 -> splitcomp_multiport/43
  ratechange_splitcomp/48 -> splitcomp_multiport/49
  ratechange_splitcomp/47 -> splitcomp_multiport/48
  ratechange_splitcomp/46 -> splitcomp_multiport/47
  splitcomp_multiport/1 -> out0/1

== system gm_Model/DUT_Test/Goertzel/EnabledGoertzel/crp_temp_streamed/counter ==
  globalSchedule : EnablePort  OutDataTypeStr=boolean
  ctr_0_47 : hdlsllib/Sources/HDL Counter  CountType=Count limited  CountInit=double(0)  CountStep=double(1)  CountMax=double(47)  CountFromType=Initial value  CountFrom=double(0)  CountResetPort=off  CountLoadPort=off  CountEnbPort=off  CountDirPort=off  CountHitOutputPort=off  CountDataType=Unsigned  CountWordLen=6  CountFracLen=0  CountSampTime=3.125e-07
  out0 : Outport  OutDataTypeStr=fixdt(0, 6, 0)  SampleTime=3.125e-07  InitialOutput=0
  wires:
  ctr_0_47/1 -> out0/1

== system gm_Model/DUT_Test/Goertzel/EnabledGoertzel/crp_temp_streamed/samples_in_bypass ==
  in0 : Inport  OutDataTypeStr=fixdt(1, 12, 11)  SampleTime=3.125e-07
  in1 : Inport  Port=2  OutDataTypeStr=boolean  SampleTime=3.125e-07
  samples_in_enb : Switch  Criteria=u2 ~= 0  Threshold=double(0)  OutDataTypeStr=fixdt(1, 12, 11)  SampleTime=3.125e-07  SaturateOnIntegerOverflow=off  InputSameDT=off
  samples_in_state : Delay  DelayLength=double(1)  InitialCondition=0  SampleTime=3.125e-07
  out0 : Outport  OutDataTypeStr=fixdt(1, 12, 11)  SampleTime=3.125e-07
  wires:
  in0/1 -> samples_in_enb/1
  in1/1 -> samples_in_enb/2
  samples_in_state/1 -> samples_in_enb/3
  samples_in_enb/1 -> samples_in_state/1, out0/1

== system gm_Model/DUT_Test/Goertzel/EnabledGoertzel/crp_temp_streamed/tappedDelay ==
  in0 : Inport  OutDataTypeStr=fixdt(1, 12, 11)  SampleTime=3.125e-07
  globalSchedule : EnablePort  OutDataTypeStr=boolean
  StateControl : StateControl  StateControl=Synchronous
  tapped_delay : simulink/Discrete/Tapped Delay  vinit=0  samptime=-1  NumDelays=double(47)  DelayOrder=Oldest  includeCurrent=off
  out0 : Outport  OutDataTypeStr=fixdt(1, 12, 11)  PortDimensions=[47]  SampleTime=3.125e-07  InitialOutput=0
  wires:
  in0/1 -> tapped_delay/1
  tapped_delay/1 -> out0/1

== system gm_Model/DUT_Test/Goertzel/EnabledGoertzel/crp_temp_streamed1/Serializer_Subnetwork ==
  in0 : Inport  OutDataTypeStr=fixdt(1, 18, 13)  PortDimensions=[1 48]  SampleTime=3.125e-07
  in1 : Inport  Port=2  OutDataTypeStr=fixdt(0, 6, 0)  SampleTime=3.125e-07
  ratechange_splitcomp : Demux  Outputs=48
  splitcomp_multiport : MultiPortSwitch  DataPortOrder=Zero-based contiguous  Inputs=48  DiagnosticForDefault=None  zeroidx=on  OutDataTypeStr=fixdt(1, 18, 13)  SampleTime=3.125e-07  SaturateOnIntegerOverflow=off  InputSameDT=off
  out0 : Outport  OutDataTypeStr=fixdt(1, 18, 13)  SampleTime=3.125e-07
  wires:
  ratechange_splitcomp/32 -> splitcomp_multiport/33
  ratechange_splitcomp/31 -> splitcomp_multiport/32
  ratechange_splitcomp/30 -> splitcomp_multiport/31
  ratechange_splitcomp/29 -> splitcomp_multiport/30
  in0/1 -> ratechange_splitcomp/1
  in1/1 -> splitcomp_multiport/1
  ratechange_splitcomp/1 -> splitcomp_multiport/2
  ratechange_splitcomp/2 -> splitcomp_multiport/3
  ratechange_splitcomp/3 -> splitcomp_multiport/4
  ratechange_splitcomp/4 -> splitcomp_multiport/5
  ratechange_splitcomp/8 -> splitcomp_multiport/9
  ratechange_splitcomp/7 -> splitcomp_multiport/8
  ratechange_splitcomp/5 -> splitcomp_multiport/6
  ratechange_splitcomp/6 -> splitcomp_multiport/7
  ratechange_splitcomp/12 -> splitcomp_multiport/13
  ratechange_splitcomp/11 -> splitcomp_multiport/12
  ratechange_splitcomp/10 -> splitcomp_multiport/11
  ratechange_splitcomp/9 -> splitcomp_multiport/10
  ratechange_splitcomp/16 -> splitcomp_multiport/17
  ratechange_splitcomp/15 -> splitcomp_multiport/16
  ratechange_splitcomp/14 -> splitcomp_multiport/15
  ratechange_splitcomp/13 -> splitcomp_multiport/14
  ratechange_splitcomp/20 -> splitcomp_multiport/21
  ratechange_splitcomp/19 -> splitcomp_multiport/20
  ratechange_splitcomp/18 -> splitcomp_multiport/19
  ratechange_splitcomp/17 -> splitcomp_multiport/18
  ratechange_splitcomp/24 -> splitcomp_multiport/25
  ratechange_splitcomp/23 -> splitcomp_multiport/24
  ratechange_splitcomp/22 -> splitcomp_multiport/23
  ratechange_splitcomp/21 -> splitcomp_multiport/22
  ratechange_splitcomp/28 -> splitcomp_multiport/29
  ratechange_splitcomp/27 -> splitcomp_multiport/28
  ratechange_splitcomp/26 -> splitcomp_multiport/27
  ratechange_splitcomp/25 -> splitcomp_multiport/26
  ratechange_splitcomp/36 -> splitcomp_multiport/37
  ratechange_splitcomp/35 -> splitcomp_multiport/36
  ratechange_splitcomp/34 -> splitcomp_multiport/35
  ratechange_splitcomp/33 -> splitcomp_multiport/34
  ratechange_splitcomp/40 -> splitcomp_multiport/41
  ratechange_splitcomp/39 -> splitcomp_multiport/40
  ratechange_splitcomp/38 -> splitcomp_multiport/39
  ratechange_splitcomp/37 -> splitcomp_multiport/38
  ratechange_splitcomp/44 -> splitcomp_multiport/45
  ratechange_splitcomp/43 -> splitcomp_multiport/44
  ratechange_splitcomp/42 -> splitcomp_multiport/43
  ratechange_splitcomp/41 -> splitcomp_multiport/42
  ratechange_splitcomp/48 -> splitcomp_multiport/49
  ratechange_splitcomp/47 -> splitcomp_multiport/48
  ratechange_splitcomp/46 -> splitcomp_multiport/47
  ratechange_splitcomp/45 -> splitcomp_multiport/46
  splitcomp_multiport/1 -> out0/1

== system gm_Model/DUT_Test/Goertzel/EnabledGoertzel/crp_temp_streamed1/Serializer_Subnetwork1 ==
  in0 : Inport  OutDataTypeStr=fixdt(1, 18, 13)  PortDimensions=[1 48]  SampleTime=3.125e-07
  in1 : Inport  Port=2  OutDataTypeStr=fixdt(0, 6, 0)  SampleTime=3.125e-07
  ratechange_splitcomp : Demux  Outputs=48
  splitcomp_multiport : MultiPortSwitch  DataPortOrder=Zero-based contiguous  Inputs=48  DiagnosticForDefault=None  zeroidx=on  OutDataTypeStr=fixdt(1, 18, 13)  SampleTime=3.125e-07  SaturateOnIntegerOverflow=off  InputSameDT=off
  out0 : Outport  OutDataTypeStr=fixdt(1, 18, 13)  SampleTime=3.125e-07
  wires:
  ratechange_splitcomp/46 -> splitcomp_multiport/47
  ratechange_splitcomp/45 -> splitcomp_multiport/46
  ratechange_splitcomp/44 -> splitcomp_multiport/45
  ratechange_splitcomp/43 -> splitcomp_multiport/44
  in0/1 -> ratechange_splitcomp/1
  ratechange_splitcomp/48 -> splitcomp_multiport/49
  ratechange_splitcomp/47 -> splitcomp_multiport/48
  in1/1 -> splitcomp_multiport/1
  ratechange_splitcomp/1 -> splitcomp_multiport/2
  ratechange_splitcomp/42 -> splitcomp_multiport/43
  ratechange_splitcomp/2 -> splitcomp_multiport/3
  ratechange_splitcomp/3 -> splitcomp_multiport/4
  ratechange_splitcomp/4 -> splitcomp_multiport/5
  ratechange_splitcomp/5 -> splitcomp_multiport/6
  ratechange_splitcomp/9 -> splitcomp_multiport/10
  ratechange_splitcomp/8 -> splitcomp_multiport/9
  ratechange_splitcomp/7 -> splitcomp_multiport/8
  ratechange_splitcomp/6 -> splitcomp_multiport/7
  ratechange_splitcomp/13 -> splitcomp_multiport/14
  ratechange_splitcomp/12 -> splitcomp_multiport/13
  ratechange_splitcomp/11 -> splitcomp_multiport/12
  ratechange_splitcomp/10 -> splitcomp_multiport/11
  ratechange_splitcomp/17 -> splitcomp_multiport/18
  ratechange_splitcomp/16 -> splitcomp_multiport/17
  ratechange_splitcomp/15 -> splitcomp_multiport/16
  ratechange_splitcomp/14 -> splitcomp_multiport/15
  ratechange_splitcomp/40 -> splitcomp_multiport/41
  ratechange_splitcomp/21 -> splitcomp_multiport/22
  ratechange_splitcomp/20 -> splitcomp_multiport/21
  ratechange_splitcomp/19 -> splitcomp_multiport/20
  ratechange_splitcomp/18 -> splitcomp_multiport/19
  ratechange_splitcomp/25 -> splitcomp_multiport/26
  ratechange_splitcomp/24 -> splitcomp_multiport/25
  ratechange_splitcomp/23 -> splitcomp_multiport/24
  ratechange_splitcomp/22 -> splitcomp_multiport/23
  ratechange_splitcomp/29 -> splitcomp_multiport/30
  ratechange_splitcomp/28 -> splitcomp_multiport/29
  ratechange_splitcomp/27 -> splitcomp_multiport/28
  ratechange_splitcomp/26 -> splitcomp_multiport/27
  ratechange_splitcomp/33 -> splitcomp_multiport/34
  ratechange_splitcomp/32 -> splitcomp_multiport/33
  ratechange_splitcomp/31 -> splitcomp_multiport/32
  ratechange_splitcomp/30 -> splitcomp_multiport/31
  ratechange_splitcomp/37 -> splitcomp_multiport/38
  ratechange_splitcomp/36 -> splitcomp_multiport/37
  ratechange_splitcomp/35 -> splitcomp_multiport/36
  ratechange_splitcomp/34 -> splitcomp_multiport/35
  ratechange_splitcomp/39 -> splitcomp_multiport/40
  ratechange_splitcomp/38 -> splitcomp_multiport/39
  ratechange_splitcomp/41 -> splitcomp_multiport/42
  splitcomp_multiport/1 -> out0/1

== system gm_Model/DUT_Test/Goertzel/EnabledGoertzel/crp_temp_streamed1/Switch_out1_bypass ==
  in0 : Inport  OutDataTypeStr=fixdt(1, 18, 13)  SampleTime=3.125e-07
  in1 : Inport  Port=2  OutDataTypeStr=boolean  SampleTime=3.125e-07
  Switch_out1_enb : Switch  Criteria=u2 ~= 0  Threshold=double(0)  OutDataTypeStr=fixdt(1, 18, 13)  SampleTime=3.125e-07  SaturateOnIntegerOverflow=off  InputSameDT=off
  Switch_out1_state : Delay  DelayLength=double(1)  InitialCondition=0  SampleTime=3.125e-07
  out0 : Outport  OutDataTypeStr=fixdt(1, 18, 13)  SampleTime=3.125e-07
  wires:
  in0/1 -> Switch_out1_enb/1
  in1/1 -> Switch_out1_enb/2
  Switch_out1_state/1 -> Switch_out1_enb/3
  Switch_out1_enb/1 -> Switch_out1_state/1, out0/1

== system gm_Model/DUT_Test/Goertzel/EnabledGoertzel/crp_temp_streamed1/counter ==
  globalSchedule : EnablePort  OutDataTypeStr=boolean
  ctr_0_47 : hdlsllib/Sources/HDL Counter  CountType=Count limited  CountInit=double(0)  CountStep=double(1)  CountMax=double(47)  CountFromType=Initial value  CountFrom=double(0)  CountResetPort=off  CountLoadPort=off  CountEnbPort=off  CountDirPort=off  CountHitOutputPort=off  CountDataType=Unsigned  CountWordLen=6  CountFracLen=0  CountSampTime=3.125e-07
  out0 : Outport  OutDataTypeStr=fixdt(0, 6, 0)  SampleTime=3.125e-07  InitialOutput=0
  wires:
  ctr_0_47/1 -> out0/1

== system gm_Model/DUT_Test/Goertzel/EnabledGoertzel/crp_temp_streamed1/tappedDelay ==
  in0 : Inport  OutDataTypeStr=fixdt(1, 18, 13)  SampleTime=3.125e-07
  globalSchedule : EnablePort  OutDataTypeStr=boolean
  StateControl : StateControl  StateControl=Synchronous
  tapped_delay : simulink/Discrete/Tapped Delay  vinit=0  samptime=-1  NumDelays=double(47)  DelayOrder=Oldest  includeCurrent=off
  out0 : Outport  OutDataTypeStr=fixdt(1, 18, 13)  PortDimensions=[47]  SampleTime=3.125e-07  InitialOutput=0
  wires:
  in0/1 -> tapped_delay/1
  tapped_delay/1 -> out0/1

== system gm_Model/DUT_Test/Goertzel/EnabledGoertzel/crp_temp_streamed2/Serializer_Subnetwork ==
  in0 : Inport  OutDataTypeStr=fixdt(1, 18, 13)  PortDimensions=[1 48]  SampleTime=3.125e-07
  in1 : Inport  Port=2  OutDataTypeStr=fixdt(0, 6, 0)  SampleTime=3.125e-07
  ratechange_splitcomp : Demux  Outputs=48
  splitcomp_multiport : MultiPortSwitch  DataPortOrder=Zero-based contiguous  Inputs=48  DiagnosticForDefault=None  zeroidx=on  OutDataTypeStr=fixdt(1, 18, 13)  SampleTime=3.125e-07  SaturateOnIntegerOverflow=off  InputSameDT=off
  out0 : Outport  OutDataTypeStr=fixdt(1, 18, 13)  SampleTime=3.125e-07
  wires:
  splitcomp_multiport/1 -> out0/1
  in0/1 -> ratechange_splitcomp/1
  in1/1 -> splitcomp_multiport/1
  ratechange_splitcomp/1 -> splitcomp_multiport/2
  ratechange_splitcomp/2 -> splitcomp_multiport/3
  ratechange_splitcomp/3 -> splitcomp_multiport/4
  ratechange_splitcomp/7 -> splitcomp_multiport/8
  ratechange_splitcomp/4 -> splitcomp_multiport/5
  ratechange_splitcomp/5 -> splitcomp_multiport/6
  ratechange_splitcomp/6 -> splitcomp_multiport/7
  ratechange_splitcomp/11 -> splitcomp_multiport/12
  ratechange_splitcomp/10 -> splitcomp_multiport/11
  ratechange_splitcomp/9 -> splitcomp_multiport/10
  ratechange_splitcomp/8 -> splitcomp_multiport/9
  ratechange_splitcomp/15 -> splitcomp_multiport/16
  ratechange_splitcomp/14 -> splitcomp_multiport/15
  ratechange_splitcomp/13 -> splitcomp_multiport/14
  ratechange_splitcomp/12 -> splitcomp_multiport/13
  ratechange_splitcomp/19 -> splitcomp_multiport/20
  ratechange_splitcomp/18 -> splitcomp_multiport/19
  ratechange_splitcomp/17 -> splitcomp_multiport/18
  ratechange_splitcomp/16 -> splitcomp_multiport/17
  ratechange_splitcomp/23 -> splitcomp_multiport/24
  ratechange_splitcomp/22 -> splitcomp_multiport/23
  ratechange_splitcomp/21 -> splitcomp_multiport/22
  ratechange_splitcomp/20 -> splitcomp_multiport/21
  ratechange_splitcomp/27 -> splitcomp_multiport/28
  ratechange_splitcomp/26 -> splitcomp_multiport/27
  ratechange_splitcomp/25 -> splitcomp_multiport/26
  ratechange_splitcomp/24 -> splitcomp_multiport/25
  ratechange_splitcomp/31 -> splitcomp_multiport/32
  ratechange_splitcomp/30 -> splitcomp_multiport/31
  ratechange_splitcomp/29 -> splitcomp_multiport/30
  ratechange_splitcomp/28 -> splitcomp_multiport/29
  ratechange_splitcomp/35 -> splitcomp_multiport/36
  ratechange_splitcomp/34 -> splitcomp_multiport/35
  ratechange_splitcomp/33 -> splitcomp_multiport/34
  ratechange_splitcomp/32 -> splitcomp_multiport/33
  ratechange_splitcomp/39 -> splitcomp_multiport/40
  ratechange_splitcomp/38 -> splitcomp_multiport/39
  ratechange_splitcomp/37 -> splitcomp_multiport/38
  ratechange_splitcomp/36 -> splitcomp_multiport/37
  ratechange_splitcomp/43 -> splitcomp_multiport/44
  ratechange_splitcomp/42 -> splitcomp_multiport/43
  ratechange_splitcomp/41 -> splitcomp_multiport/42
  ratechange_splitcomp/40 -> splitcomp_multiport/41
  ratechange_splitcomp/47 -> splitcomp_multiport/48
  ratechange_splitcomp/46 -> splitcomp_multiport/47
  ratechange_splitcomp/45 -> splitcomp_multiport/46
  ratechange_splitcomp/44 -> splitcomp_multiport/45
  ratechange_splitcomp/48 -> splitcomp_multiport/49
